simulink model "Squaring_Loop_Demodulator"  (R2013a)
settings: Solver=ode3  SolverMode=SingleTasking  StartTime=0.0  StopTime=1  FixedStep=1/480e3  RelTol=1e-3
libraries: dsparch4 x4, commfilt2 x2, commrandsrc2 x1, commchan3 x1, simulink x1, simulink_extras x1, commsynccomp2 x1, commsink2 x1
settings Model: Creator=tibbs2010  LastModifiedBy=tibbs2010

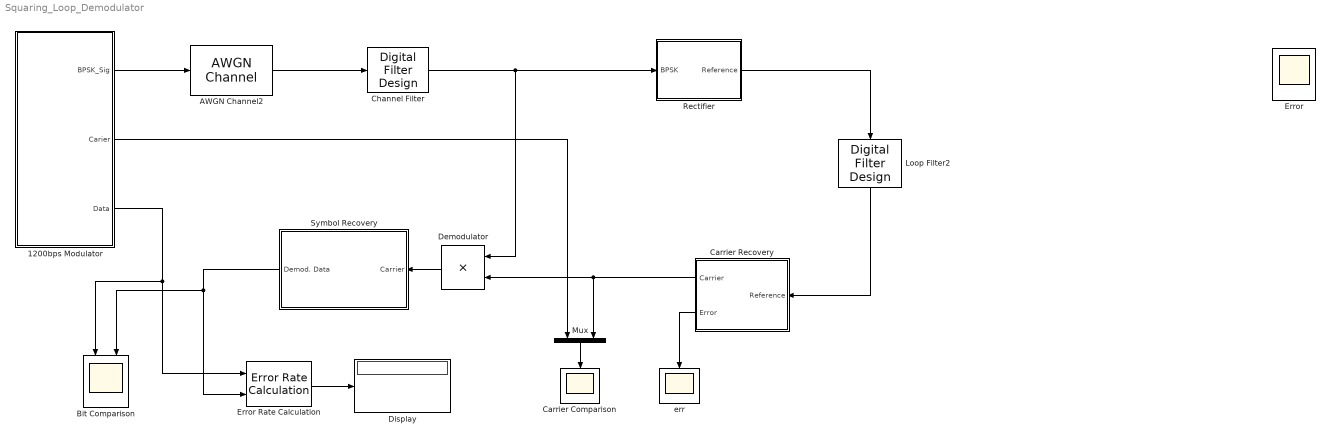
== system Squaring_Loop_Demodulator ==
  1200bps Modulator : Subsystem
  AWGN Channel2 : commchan3/AWGN Channel  InputProcessing=Columns as channels (frame based)  seed=randseed  noiseMode="Signal to noise ratio  (Eb/No)"  EbNodB=8  EsNodB=10  SNRdB=10  bitsPerSym=1  Ps=12.5  Tsym=1/1200  variance=1
  Bit Comparison : Scope  NumInputPorts=2
      settings: YMin=-0.5~-0.5  YMax=1.5~1.5
  Carrier Comparison : Scope
      settings: YMin=-5.5  YMax=5.5  SaveName=ScopeData2
  Carrier Recovery : Subsystem
  Channel Filter : dsparch4/Digital Filter Design  mwdsp_browser_bugfix_var=off
  Demodulator : Product
  Display : Display
  Error : Scope
      settings: YMin=-0.4  YMax=0.45
  Error Rate Calculation : commsink2/Error Rate Calculation  N=1  st_delay=0  cp_mode=Entire frame  subframe=[]  PMode=Port  WsName=ErrorVec  RsMode2=off  stop=off  numErr=100  maxBits=1e6
  Loop Filter2 : dsparch4/Digital Filter Design  mwdsp_browser_bugfix_var=off
  Mux : Mux  Inputs=2
  Rectifier : Subsystem
  Symbol Recovery : Subsystem
  err : Scope
      settings: TimeRange=0.002527976522640303  YMin=-8  YMax=8  SaveName=ScopeData3
  wires:
  Mux/1 -> Carrier Comparison/1
  Carrier Recovery/1(Carrier) -> Mux/2, Demodulator/2
  Demodulator/1 -> Symbol Recovery/1(Carrier)
  Symbol Recovery/1(Demod. Data) -> Bit Comparison/2, Error Rate Calculation/2
  1200bps Modulator/3(Data) -> Bit Comparison/1, Error Rate Calculation/1
  Error Rate Calculation/1 -> Display/1
  Carrier Recovery/2(Error) -> err/1
  1200bps Modulator/2(Carier) -> Mux/1
  Rectifier/1(Reference) -> Loop Filter2/1
  Loop Filter2/1 -> Carrier Recovery/1(Reference)
  1200bps Modulator/1(BPSK_Sig) -> AWGN Channel2/1
  Channel Filter/1 -> Demodulator/1, Rectifier/1(BPSK)
  AWGN Channel2/1 -> Channel Filter/1

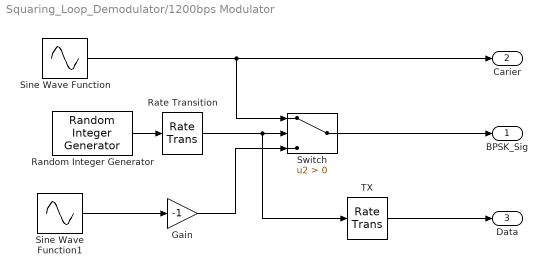
== system Squaring_Loop_Demodulator/1200bps Modulator ==
  Gain : Gain  Gain=-1
  Random Integer Generator : commrandsrc2/Random Integer Generator  mul=2  seed=randseed  Ts=1/1200  frameBased=off  sampPerFrame=1  orient=off  outDataType=double
  Rate Transition : RateTransition  OutPortSampleTime=1/480e3
  Sine Wave Function : Sin  Amplitude=5  Frequency=2*pi*2400  SampleTime=1/480e3
  Sine Wave Function1 : Sin  Amplitude=5  Frequency=2*pi*2400  SampleTime=1/480e3
  Switch : Switch  Criteria=u2 > Threshold
  TX : RateTransition  OutPortSampleTime=1/1200
  BPSK_Sig : Outport
  Carier : Outport  Port=2
  Data : Outport  Port=3
  wires:
  Random Integer Generator/1 -> Rate Transition/1
  Rate Transition/1 -> TX/1, Switch/2
  Sine Wave Function/1 -> Carier/1, Switch/1
  Sine Wave Function1/1 -> Gain/1
  Gain/1 -> Switch/3
  Switch/1 -> BPSK_Sig/1
  TX/1 -> Data/1

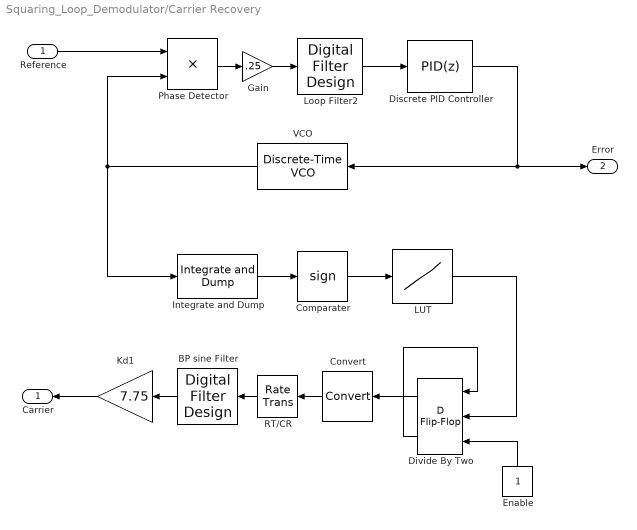
== system Squaring_Loop_Demodulator/Carrier Recovery ==
  Reference : Inport
  BP sine Filter : dsparch4/Digital Filter Design  mwdsp_browser_bugfix_var=off
  Comparater : Signum
  Convert : DataTypeConversion
  Discrete PID Controller : simulink/Continuous/PID Controller  Controller=PID  TimeDomain=Discrete-time  SampleTime=1/480e3  IntegratorMethod=Forward Euler  FilterMethod=Forward Euler  Form=Parallel  P=1  I=10  D=3  N=1  InitialConditionSource=internal  InitialConditionForIntegrator=0  InitialConditionForFilter=0  ExternalReset=none  LimitOutput=off  UpperSaturationLimit=inf  LowerSaturationLimit=-inf  LinearizeAsGain=off  AntiWindupMode=none  Kb=1  TrackingMode=off  Kt=1  PParamMin=[]  PParamMax=[]  IParamMin=[]  IParamMax=[]  DParamMin=[]  DParamMax=[]  NParamMin=[]  NParamMax=[]  KbParamMin=[]  KbParamMax=[]  KtParamMin=[]  KtParamMax=[]  POutMin=[]  POutMax=[]  IOutMin=[]  IOutMax=[]  DOutMin=[]  DOutMax=[]  NOutMin=[]  NOutMax=[]  KbOutMin=[]  KbOutMax=[]  KtOutMin=[]  KtOutMax=[]  IntegratorOutMin=[]  IntegratorOutMax=[]  FilterOutMin=[]  FilterOutMax=[]  SumOutMin=[]  SumOutMax=[]  SumI1OutMin=[]  SumI1OutMax=[]  SumI2OutMin=[]  SumI2OutMax=[]  SumI3OutMin=[]  SumI3OutMax=[]  SumDOutMin=[]  SumDOutMax=[]  SaturationOutMin=[]  SaturationOutMax=[]  IntegratorContinuousStateAttributes=''  IntegratorStateMustResolveToSignalObject=off  IntegratorRTWStateStorageClass=Auto  FilterContinuousStateAttributes=''  FilterStateMustResolveToSignalObject=off  FilterRTWStateStorageClass=Auto
  Divide By Two : simulink_extras/Flip Flops/D Flip-Flop
  Enable : Constant
  Gain : Gain  Gain=.25
  Integrate and Dump : commfilt2/Integrate and Dump  obssamples=50  offsetsamples=0  nodump=off  roundingMode=Floor  overflowMode=off
  Kd1 : Gain  Gain=7.75
  LUT : Lookup_n-D  NumberOfTableDimensions=1  BreakpointsForDimension1=[-1 0 1]  Table=[0 0 1]  RndMeth=Simplest  InputSameDT=on
  Loop Filter2 : dsparch4/Digital Filter Design  mwdsp_browser_bugfix_var=off
  Phase Detector : Product
  RT/CR : RateTransition  OutPortSampleTime=1/480e3
  VCO : commsynccomp2/Discrete-Time VCO  Ac=5  Fc=4800  Kc=1  Ph=pi  ts=1/480e3
  Carrier : Outport
  Error : Outport  Port=2
  wires:
  Kd1/1 -> Carrier/1
  Convert/1 -> RT/CR/1
  RT/CR/1 -> BP sine Filter/1
  Comparater/1 -> LUT/1
  Enable/1 -> Divide By Two/3
  Integrate and Dump/1 -> Comparater/1
  Divide By Two/1 -> Convert/1
  VCO/1 -> Phase Detector/2, Integrate and Dump/1
  Reference/1 -> Phase Detector/1
  BP sine Filter/1 -> Kd1/1
  LUT/1 -> Divide By Two/2
  Divide By Two/2 -> Divide By Two/1
  Loop Filter2/1 -> Discrete PID Controller/1
  Phase Detector/1 -> Gain/1
  Discrete PID Controller/1 -> Error/1, VCO/1
  Gain/1 -> Loop Filter2/1

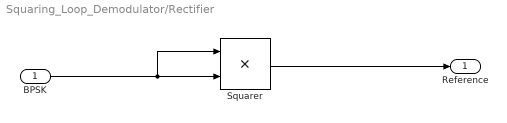
== system Squaring_Loop_Demodulator/Rectifier ==
  BPSK : Inport
  Squarer : Product
  Reference : Outport
  wires:
  BPSK/1 -> Squarer/2, Squarer/1
  Squarer/1 -> Reference/1

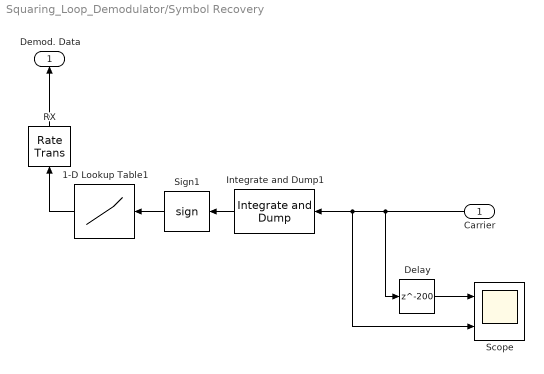
== system Squaring_Loop_Demodulator/Symbol Recovery ==
  Carrier : Inport
  1-D Lookup Table1 : Lookup_n-D  NumberOfTableDimensions=1  BreakpointsForDimension1=[-1 0 1]  Table=[0 0 1]  RndMeth=Simplest  InputSameDT=on
  Delay : Delay  DelayLength=200  InitialCondition=0
  Integrate and Dump1 : commfilt2/Integrate and Dump  obssamples=400  offsetsamples=0  nodump=off  roundingMode=Floor  overflowMode=off
  RX : RateTransition  OutPortSampleTime=1/1200
  Scope : Scope  NumInputPorts=2
      settings: YMin=-5~-5  YMax=5~5  SaveName=ScopeData4
  Sign1 : Signum
  Demod. Data : Outport
  wires:
  RX/1 -> Demod. Data/1
  Sign1/1 -> 1-D Lookup Table1/1
  Carrier/1 -> Delay/1, Scope/2, Integrate and Dump1/1
  1-D Lookup Table1/1 -> RX/1
  Integrate and Dump1/1 -> Sign1/1
  Delay/1 -> Scope/1
